simulink model "test"  (R2024b)
settings: Solver=VariableStepAuto  StartTime=0.0  StopTime=T_s  RelTol=1e-3
values from neighbouring files (symbols this model uses):
  atan_scale = 100    [Exercise_1_done.mat]
  b_1 = 0.00287081256979    [Exercise_1_done.mat]
  b_2 = 0.000164101446955    [Exercise_1_done.mat]
  b_3 = 0.000179179608867    [Exercise_1_done.mat]
  J_1 = 0.00238607064451    [Exercise_1_done.mat]
  J_2 = 0.00182883419357    [Exercise_1_done.mat]
  J_3 = 0.00182883419357    [Exercise_1_done.mat]
  k_1 = 2.78736928639    [Exercise_1_done.mat]
  k_2 = 2.53389832968    [Exercise_1_done.mat]
  T_Cm = 0.0969711017207    [Exercise_1_done.mat]
  T_Cp = 0.0714454263135    [Exercise_1_done.mat]
  w_th = 0.75    [Exercise_1_done.mat]
  x_0 = [0 0 0 0 0 0]    [Exercise_1_done.mat]
settings Model: Creator=lukas  LastModifiedBy=lukas

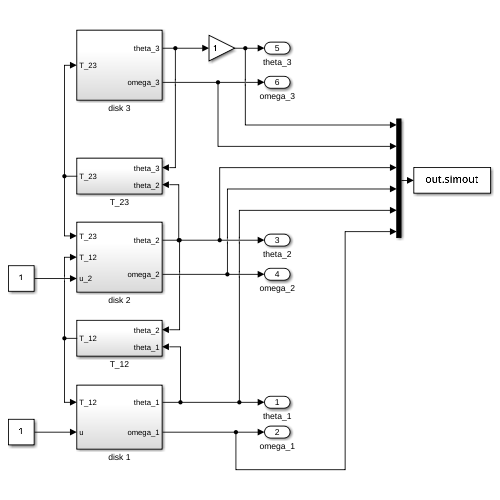
[thumbnail: Simulink's stored preview of the top-level diagram]
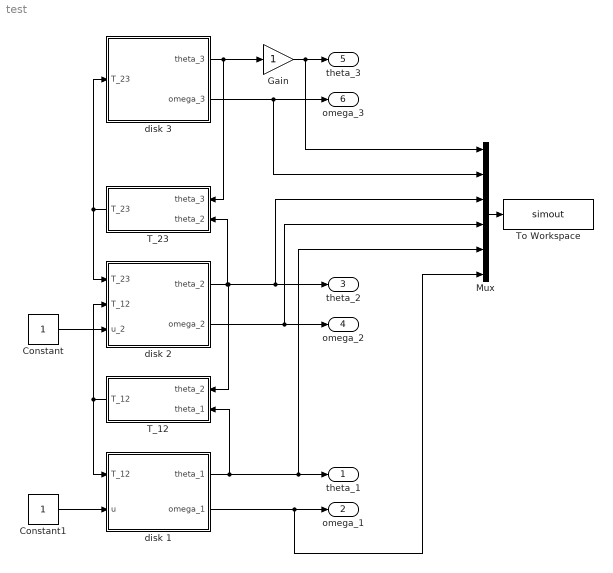
== system test ==
  Constant : Constant
  Constant1 : Constant
  Gain : Gain
  Mux : Mux  Inputs=6
  T_12 : Subsystem
  T_23 : Subsystem
  To Workspace : ToWorkspace  VariableName=simout  SaveFormat=Timeseries  SampleTime=-1
  disk 1 : Subsystem
  disk 2 : Subsystem
  disk 3 : Subsystem
  theta_1 : Outport  VectorParamsAs1DForOutWhenUnconnected=off
  omega_1 : Outport  Port=2  VectorParamsAs1DForOutWhenUnconnected=off
  theta_2 : Outport  Port=3  VectorParamsAs1DForOutWhenUnconnected=off
  omega_2 : Outport  Port=4  VectorParamsAs1DForOutWhenUnconnected=off
  theta_3 : Outport  Port=5  VectorParamsAs1DForOutWhenUnconnected=off
  omega_3 : Outport  Port=6  VectorParamsAs1DForOutWhenUnconnected=off
  wires:
  disk 2/1(theta_2) -> T_23/2(theta_2), Mux/3, theta_2/1, T_12/1(theta_2)
  disk 1/1(theta_1) -> Mux/5, theta_1/1, T_12/2(theta_1)
  T_23/1(T_23) -> disk 2/1(T_23), disk 3/1(T_23)
  disk 1/2(omega_1) -> Mux/6, omega_1/1
  Constant1/1 -> disk 1/2(u)
  disk 2/2(omega_2) -> Mux/4, omega_2/1
  disk 3/1(theta_3) -> Gain/1, T_23/1(theta_3)
  T_12/1(T_12) -> disk 1/1(T_12), disk 2/2(T_12)
  Constant/1 -> disk 2/3(u_2)
  disk 3/2(omega_3) -> Mux/2, omega_3/1
  Gain/1 -> Mux/1, theta_3/1
  Mux/1 -> To Workspace/1

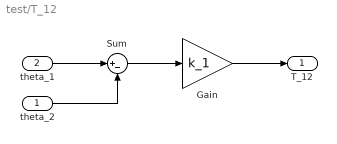
== system test/T_12 ==
  theta_2 : Inport
  theta_1 : Inport  Port=2
  Gain : Gain  Gain=k_1
  Sum : Sum  Inputs=|+-
  T_12 : Outport  VectorParamsAs1DForOutWhenUnconnected=off
  wires:
  theta_2/1 -> Sum/2
  theta_1/1 -> Sum/1
  Sum/1 -> Gain/1
  Gain/1 -> T_12/1

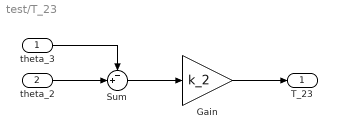
== system test/T_23 ==
  theta_3 : Inport
  theta_2 : Inport  Port=2
  Gain : Gain  Gain=k_2
  Sum : Sum  Inputs=-+|
  T_23 : Outport  VectorParamsAs1DForOutWhenUnconnected=off
  wires:
  Gain/1 -> T_23/1
  Sum/1 -> Gain/1
  theta_3/1 -> Sum/1
  theta_2/1 -> Sum/2

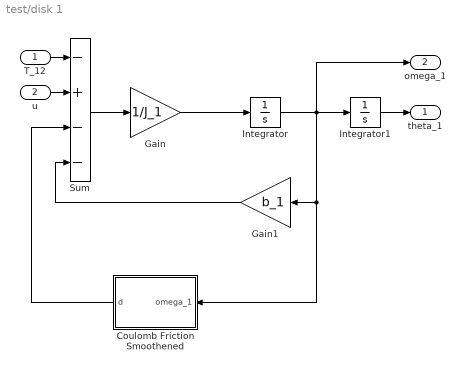
== system test/disk 1 ==
  T_12 : Inport
  u : Inport  Port=2
  Coulomb Friction Smoothened : Subsystem
  Gain : Gain  Gain=1/J_1
  Gain1 : Gain  Gain=b_1
  Integrator : Integrator  InitialCondition=x_0(2)
  Integrator1 : Integrator  InitialCondition=x_0(1)
  Sum : Sum  Inputs=-+--
  theta_1 : Outport  VectorParamsAs1DForOutWhenUnconnected=off
  omega_1 : Outport  Port=2  VectorParamsAs1DForOutWhenUnconnected=off
  wires:
  Sum/1 -> Gain/1
  Integrator/1 -> Integrator1/1, omega_1/1, Coulomb Friction Smoothened/1(omega_1), Gain1/1
  Gain1/1 -> Sum/4
  Integrator1/1 -> theta_1/1
  T_12/1 -> Sum/1
  u/1 -> Sum/2
  Gain/1 -> Integrator/1
  Coulomb Friction Smoothened/1(d) -> Sum/3

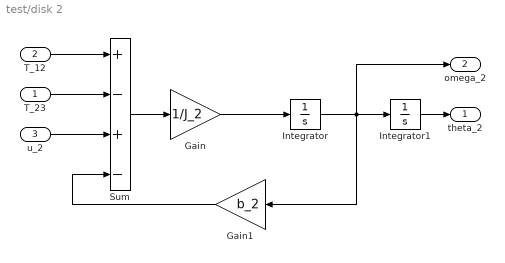
== system test/disk 2 ==
  T_23 : Inport
  T_12 : Inport  Port=2
  u_2 : Inport  Port=3
  Gain : Gain  Gain=1/J_2
  Gain1 : Gain  Gain=b_2
  Integrator : Integrator  InitialCondition=x_0(4)
  Integrator1 : Integrator  InitialCondition=x_0(3)
  Sum : Sum  Inputs=+-+-
  theta_2 : Outport  VectorParamsAs1DForOutWhenUnconnected=off
  omega_2 : Outport  Port=2  VectorParamsAs1DForOutWhenUnconnected=off
  wires:
  T_23/1 -> Sum/2
  T_12/1 -> Sum/1
  Integrator1/1 -> theta_2/1
  Gain1/1 -> Sum/4
  Gain/1 -> Integrator/1
  Integrator/1 -> Integrator1/1, Gain1/1, omega_2/1
  Sum/1 -> Gain/1
  u_2/1 -> Sum/3

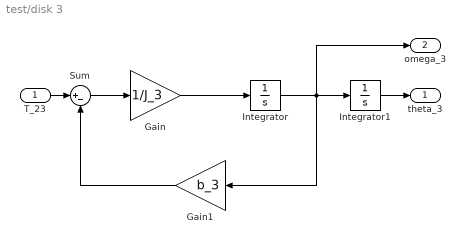
== system test/disk 3 ==
  T_23 : Inport
  Gain : Gain  Gain=1/J_3
  Gain1 : Gain  Gain=b_3
  Integrator : Integrator  InitialCondition=x_0(6)
  Integrator1 : Integrator  InitialCondition=x_0(5)
  Sum : Sum  Inputs=|+-
  theta_3 : Outport  VectorParamsAs1DForOutWhenUnconnected=off
  omega_3 : Outport  Port=2  VectorParamsAs1DForOutWhenUnconnected=off
  wires:
  Sum/1 -> Gain/1
  Integrator/1 -> Integrator1/1, omega_3/1, Gain1/1
  Gain/1 -> Integrator/1
  Gain1/1 -> Sum/2
  Integrator1/1 -> theta_3/1
  T_23/1 -> Sum/1

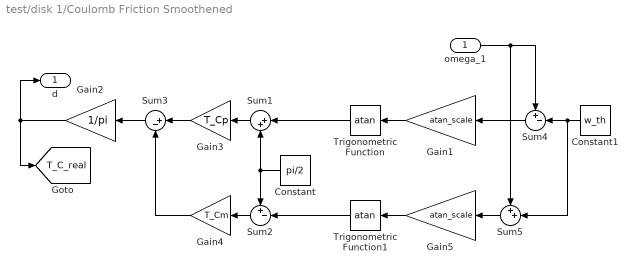
== system test/disk 1/Coulomb Friction Smoothened ==
  omega_1 : Inport
  Constant : Constant  Value=pi/2
  Constant1 : Constant  Value=w_th
  Gain1 : Gain  Gain=atan_scale
  Gain2 : Gain  Gain=1/pi
  Gain3 : Gain  Gain=T_Cp
  Gain4 : Gain  Gain=T_Cm
  Gain5 : Gain  Gain=atan_scale
  Sum1 : Sum  Inputs=|++
  Sum2 : Sum  Inputs=+-|
  Sum3 : Sum  Inputs=|+-
  Sum4 : Sum  Inputs=+-|
  Sum5 : Sum  Inputs=++|
  Trigonometric Function : Trigonometry  Operator=atan
  Trigonometric Function1 : Trigonometry  Operator=atan
  d : Outport  VectorParamsAs1DForOutWhenUnconnected=off
  tag scope: T_C_real=global
  wires:
  Gain1/1 -> Trigonometric Function/1
  Sum1/1 -> Gain3/1
  Constant/1 -> Sum2/1, Sum1/2
  Sum2/1 -> Gain4/1
  Sum3/1 -> Gain2/1
  Trigonometric Function/1 -> Sum1/1
  Gain4/1 -> Sum3/2
  Gain2/1 -> [T_C_real], d/1
  omega_1/1 -> Sum5/1, Sum4/1
  Gain3/1 -> Sum3/1
  Sum4/1 -> Gain1/1
  Constant1/1 -> Sum5/2, Sum4/2
  Gain5/1 -> Trigonometric Function1/1
  Sum5/1 -> Gain5/1
  Trigonometric Function1/1 -> Sum2/2
